simulink model "Powertrain_Simulation_2017a"  (R2017a)
settings: Solver=FixedStepAuto  StartTime=0.0  StopTime=Inf  MinStep=0.01  RelTol=1e-3
undefined symbols (not defined in the file or in its folder): A1, AIR, C1, C2, COOLANT, cp, Elevation_Profile, EM, flowrate, hA1, k12, M, M2, MOT, RAD, Velocity_Profile
libraries: simulink x5
(part 2 of 2)

== system Powertrain_Simulation_2017a/Motorcycle Model/Powertrain/Powertrain Thermal Model/Reinhardt Inverter Thermal Model/Inverter Thermal Model/Coolant Temp ==
  Module Case Temp : Inport
  Module Case Temp1 : Inport  Port=2
  Gain : Gain  Gain=hA1/(flowrate*cp)
  Sum : Sum  Inputs=+-
  Sum1 : Sum  Inputs=|++
  Electrical Device Temps : Outport
  wires:
  Module Case Temp/1 -> Sum/1  "Module Case Temp"
  Sum1/1 -> Electrical Device Temps/1  "Coolant Temp, out"
  Module Case Temp1/1 -> Sum1/2, Sum/2  "Coolant Temp, in"
  Sum/1 -> Gain/1
  Gain/1 -> Sum1/1

== system Powertrain_Simulation_2017a/Motorcycle Model/Powertrain/Powertrain Thermal Model/Reinhardt Inverter Thermal Model/Inverter Thermal Model/Inverter Electrical Devices ==
  Heat Rejection : Inport
  Module Case Temp : Inport  Port=2
  In1 : Inport  Port=3
  Gain : Gain  Gain=1/(M*C1)
  Gain1 : Gain  Gain=k12
  Integrator : Integrator
  Sum : Sum  Inputs=+-
  Sum1 : Sum  Inputs=+-
  Electrical Device Temps : Outport
  wires:
  Heat Rejection/1 -> Sum/1  "Heat Rejection"
  Module Case Temp/1 -> Sum1/1  "Electrical Device Temps"
  Integrator/1 -> Electrical Device Temps/1  "Electrical Device Temps"
  In1/1 -> Sum1/2  "Module Case Temp"
  Sum/1 -> Gain/1
  Sum1/1 -> Gain1/1
  Gain1/1 -> Sum/2
  Gain/1 -> Integrator/1  "dT1/dt"

== system Powertrain_Simulation_2017a/Motorcycle Model/Powertrain/Powertrain Thermal Model/Reinhardt Inverter Thermal Model/Inverter Thermal Model/Module Case Temp ==
  Heat Rejection : Inport
  Module Case Temp : Inport  Port=2
  Module Case Temp1 : Inport  Port=3
  Gain1 : Gain  Gain=k12
  Gain2 : Gain  Gain=h*A1
  Gain3 : Gain  Gain=1/(M2*C2)
  Integrator : Integrator
  Sum1 : Sum  Inputs=+-
  Sum2 : Sum  Inputs=+-
  Sum3 : Sum  Inputs=+-
  Electrical Device Temps : Outport
  wires:
  Integrator/1 -> Electrical Device Temps/1  "Module Case Temp"
  Module Case Temp1/1 -> Sum2/2  "Coolant Temp, in"
  Sum1/1 -> Gain1/1
  Heat Rejection/1 -> Sum1/1  "Electrical Device Temp"
  Gain1/1 -> Sum3/1
  Module Case Temp/1 -> Sum2/1, Sum1/2  "Module Case Temp"
  Sum2/1 -> Gain2/1
  Gain2/1 -> Sum3/2
  Sum3/1 -> Gain3/1
  Gain3/1 -> Integrator/1  "dT2/dt"

== system Powertrain_Simulation_2017a/Motorcycle Model/Powertrain/Powertrain Thermal Model/Radiator Thermal Model/Reduced Radiator Thermal Model (1 Node - 1 Mass)/Node 1/Convection Coefficient (Coolant Side) ==
  q_c : Inport
  Constant1 : Constant  Value=RAD.beta
  Constant2 : Constant  Value=1/3
  Constant3 : Constant  Value=RAD.beta
  Constant4 : Constant  Value=RAD.C3
  Divide : Product  Inputs=**/
  Divide1 : Product  Inputs=**
  Divide4 : Product  Inputs=**/
  Math Function1 : Math  Operator=pow  SaturateOnIntegerOverflow=on
  Math Function2 : Math  Operator=pow  SaturateOnIntegerOverflow=on
  Math Function3 : Math  Operator=pow  SaturateOnIntegerOverflow=on
  C_conv : Outport
  wires:
  Math Function3/1 -> Divide/3
  [mu_cool] -> Math Function3/1
  Constant3/1 -> Math Function3/2
  Math Function1/1 -> Divide/1
  Constant2/1 -> Math Function1/2
  Math Function2/1 -> Divide4/2
  Divide1/1 -> Math Function2/1
  Constant1/1 -> Math Function2/2
  [k_cool] -> Divide/2
  [Pr_cool] -> Math Function1/1
  [rho_cool] -> Divide1/1
  q_c/1 -> Divide1/2
  Constant4/1 -> Divide4/3
  Divide/1 -> Divide4/1  "Cf"
  Divide4/1 -> C_conv/1

== system Powertrain_Simulation_2017a/Motorcycle Model/Powertrain/Powertrain Thermal Model/Radiator Thermal Model/Reduced Radiator Thermal Model (1 Node - 1 Mass)/Node 1/Fins Thermal Mass ==
  Constant1 : Constant  Value=(RAD.delt * RAD.dc * RAD.Lf) / (RAD.St * RAD.df)
  Constant2 : Constant  Value=RAD.rho_metal
  Constant4 : Constant  Value=RAD.cp_metal
  Divide4 : Product  Inputs=***
  C''s : Outport
  wires:
  Divide4/1 -> C''s/1
  Constant2/1 -> Divide4/3
  Constant4/1 -> Divide4/2
  Constant1/1 -> Divide4/1

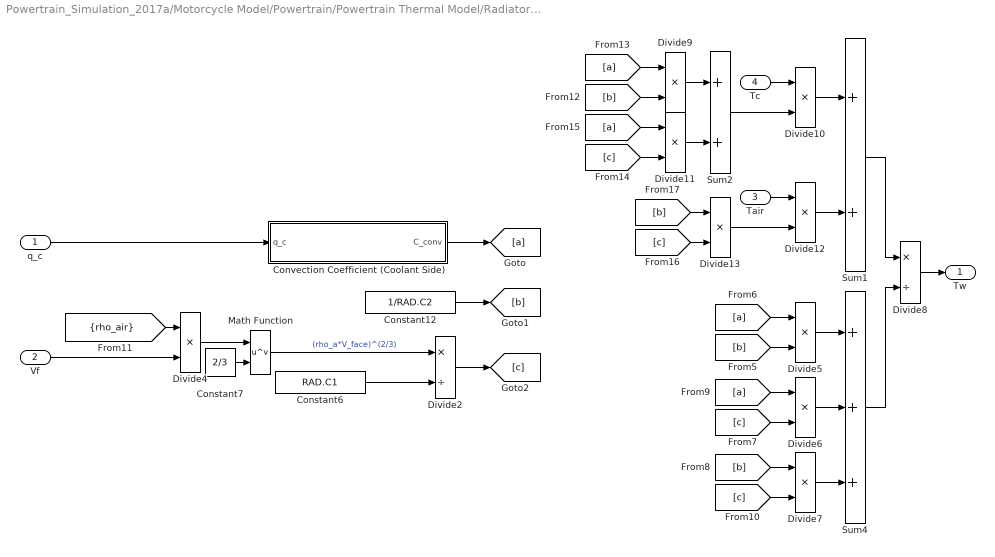
== system Powertrain_Simulation_2017a/Motorcycle Model/Powertrain/Powertrain Thermal Model/Radiator Thermal Model/Reduced Radiator Thermal Model (1 Node - 1 Mass)/Node 1/Singular Perturbation Model ==
  q_c : Inport
  Vf : Inport  Port=2
  Tair : Inport  Port=3
  Tc : Inport  Port=4
  Constant12 : Constant  Value=1/RAD.C2
  Constant6 : Constant  Value=RAD.C1
  Constant7 : Constant  Value=2/3
  Convection Coefficient (Coolant Side) : Subsystem
  Divide{4..7,9..13} (9 alike) : Product  Inputs=**
  Divide2 : Product  Inputs=*/
  Divide8 : Product  Inputs=*/
  Math Function : Math  Operator=pow  SaturateOnIntegerOverflow=on
  Sum1 : Sum
  Sum2 : Sum
  Sum4 : Sum  Inputs=+++
  Tw : Outport
  wires:
  Divide2/1 -> [c]
  Convection Coefficient (Coolant Side)/1(C_conv) -> [a]
  Constant12/1 -> [b]
  q_c/1 -> Convection Coefficient (Coolant Side)/1(q_c)
  Sum2/1 -> Divide10/2
  Divide11/1 -> Sum2/2
  Divide9/1 -> Sum2/1
  [c] -> Divide11/2
  [a] -> Divide11/1
  Tc/1 -> Divide10/1
  Divide10/1 -> Sum1/1
  Tair/1 -> Divide12/1
  [b] -> Divide9/2
  [a] -> Divide9/1
  Divide13/1 -> Divide12/2
  [c] -> Divide13/2
  [b] -> Divide13/1
  Divide12/1 -> Sum1/2
  Sum1/1 -> Divide8/1
  Sum4/1 -> Divide8/2
  Divide7/1 -> Sum4/3
  Divide6/1 -> Sum4/2
  Divide5/1 -> Sum4/1
  [c] -> Divide7/2
  [b] -> Divide7/1
  [c] -> Divide6/2
  [a] -> Divide6/1
  [b] -> Divide5/2
  [a] -> Divide5/1
  Divide4/1 -> Math Function/1
  Constant7/1 -> Math Function/2
  Math Function/1 -> Divide2/1  "(rho_a*V_face)^(2/3)"
  Constant6/1 -> Divide2/2
  [rho_air] -> Divide4/1
  Vf/1 -> Divide4/2
  Divide8/1 -> Tw/1

== system Powertrain_Simulation_2017a/Motorcycle Model/Powertrain/Powertrain Thermal Model/Radiator Thermal Model/Reduced Radiator Thermal Model (1 Node - 1 Mass)/Node 1/Wall Thermal Mass ==
  Constant1 : Constant  Value=RAD.St*( (RAD.dt - RAD.tt)*(RAD.tt - RAD.b) + pi/4*(RAD.dt^2 - RAD.b^2) )  VectorParams1D=off
  Constant2 : Constant  Value=RAD.rho_metal
  Constant4 : Constant  Value=RAD.cp_metal
  Divide4 : Product  Inputs=***
  Cw : Outport
  wires:
  Constant1/1 -> Divide4/1
  Constant4/1 -> Divide4/2
  Constant2/1 -> Divide4/3
  Divide4/1 -> Cw/1

== system Powertrain_Simulation_2017a/Motorcycle Model/Powertrain/Powertrain Thermal Model/Radiator Thermal Model/Reduced Radiator Thermal Model (1 Node - 1 Mass)/Node 1/Singular Perturbation Model/Convection Coefficient (Coolant Side) ==
  q_c : Inport
  Constant1 : Constant  Value=RAD.beta
  Constant2 : Constant  Value=1/3
  Constant3 : Constant  Value=RAD.beta
  Constant4 : Constant  Value=RAD.C3
  Divide : Product  Inputs=**/
  Divide1 : Product  Inputs=**
  Divide4 : Product  Inputs=**/
  Math Function1 : Math  Operator=pow  SaturateOnIntegerOverflow=on
  Math Function2 : Math  Operator=pow  SaturateOnIntegerOverflow=on
  Math Function3 : Math  Operator=pow  SaturateOnIntegerOverflow=on
  C_conv : Outport
  wires:
  Math Function3/1 -> Divide/3
  [mu_cool] -> Math Function3/1
  Constant3/1 -> Math Function3/2
  Math Function1/1 -> Divide/1
  Constant2/1 -> Math Function1/2
  Math Function2/1 -> Divide4/2
  Divide1/1 -> Math Function2/1
  Constant1/1 -> Math Function2/2
  [k_cool] -> Divide/2
  [Pr_cool] -> Math Function1/1
  [rho_cool] -> Divide1/1
  q_c/1 -> Divide1/2
  Constant4/1 -> Divide4/3
  Divide/1 -> Divide4/1  "Cf"
  Divide4/1 -> C_conv/1
